simulink model "Week3Problem2"  (R2020a)
settings: Solver=VariableStepAuto  StartTime=0.0  StopTime=10.0  RelTol=1e-3
settings Model: Creator=sreeram  LastModifiedBy=sreeram

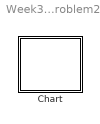
== system Week3Problem2 ==
  Chart : Stateflow chart  TreatAsAtomicUnit=on

== stateflow chart Week3Problem2/Chart ==
